simulink model "BPedalOverlap"  (R2024b)
settings: configuration reference "STM32H7_Config" (kept outside this file)
undefined symbols (not defined in the file): pBrakeOverlapThreshold, rThrottleOverlapThreshold, tSystemsTask
libraries: simulink x2
settings Model: DataDictionary=Master_Dictionary.sldd  EnableAccessToBaseWorkspace=off  Creator=torni  LastModifiedBy=William
settings ConfigSetRef: SourceName=STM32H7_Config

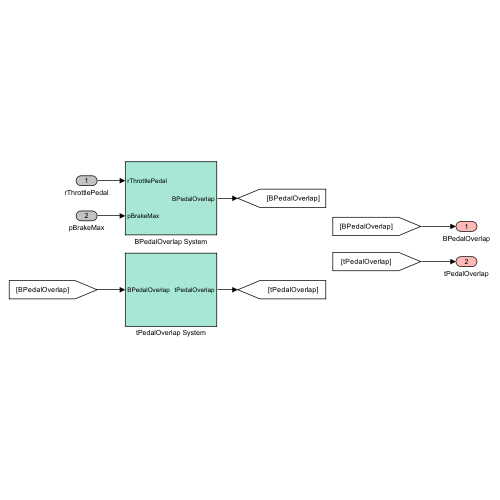
[thumbnail: Simulink's stored preview of the top-level diagram]
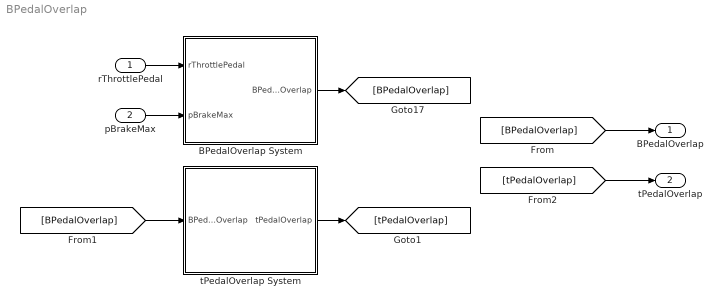
== system BPedalOverlap ==
  rThrottlePedal : Inport  OutDataTypeStr=double
  pBrakeMax : Inport  Port=2  OutDataTypeStr=double
  BPedalOverlap System : Subsystem
  tPedalOverlap System : Subsystem
  BPedalOverlap : Outport  OutDataTypeStr=boolean  VectorParamsAs1DForOutWhenUnconnected=off
  tPedalOverlap : Outport  Port=2  OutDataTypeStr=double  VectorParamsAs1DForOutWhenUnconnected=off
  wires:
  rThrottlePedal/1 -> BPedalOverlap System/1(rThrottlePedal)
  pBrakeMax/1 -> BPedalOverlap System/2(pBrakeMax)
  BPedalOverlap System/1(BPedalOverlap) -> [BPedalOverlap]
  [BPedalOverlap] -> BPedalOverlap/1
  [BPedalOverlap] -> tPedalOverlap System/1(BPedalOverlap)
  tPedalOverlap System/1(tPedalOverlap) -> [tPedalOverlap]
  [tPedalOverlap] -> tPedalOverlap/1

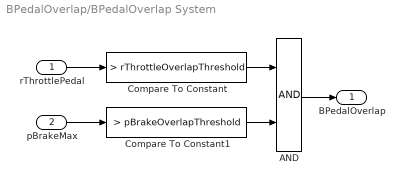
== system BPedalOverlap/BPedalOverlap System ==
  rThrottlePedal : Inport  OutDataTypeStr=double
  pBrakeMax : Inport  Port=2  OutDataTypeStr=double
  AND : Logic  AllPortsSameDT=off  OutDataTypeStr=boolean
  Compare To Constant : simulink/Logic and Bit Operations/Compare To Constant  relop=>  const=rThrottleOverlapThreshold  OutDataTypeStr=boolean
  Compare To Constant1 : simulink/Logic and Bit Operations/Compare To Constant  relop=>  const=pBrakeOverlapThreshold  OutDataTypeStr=boolean
  BPedalOverlap : Outport  OutDataTypeStr=boolean  VectorParamsAs1DForOutWhenUnconnected=off
  wires:
  Compare To Constant1/1 -> AND/2
  rThrottlePedal/1 -> Compare To Constant/1
  Compare To Constant/1 -> AND/1
  AND/1 -> BPedalOverlap/1
  pBrakeMax/1 -> Compare To Constant1/1

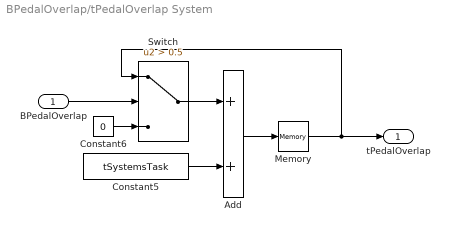
== system BPedalOverlap/tPedalOverlap System ==
  BPedalOverlap : Inport  OutDataTypeStr=boolean
  Add : Sum
  Constant5 : Constant  Value=tSystemsTask
  Constant6 : Constant  Value=0
  Memory : Memory  InheritSampleTime=on
  Switch : Switch  Criteria=u2 > Threshold  Threshold=0.5  SaturateOnIntegerOverflow=off  InputSameDT=off
  tPedalOverlap : Outport  OutDataTypeStr=double  VectorParamsAs1DForOutWhenUnconnected=off
  wires:
  Constant6/1 -> Switch/3
  Add/1 -> Memory/1
  Constant5/1 -> Add/2
  Memory/1 -> tPedalOverlap/1, Switch/1
  Switch/1 -> Add/1
  BPedalOverlap/1 -> Switch/2
